simulink model "TPS"  (R2023b)
settings: Solver=FixedStepDiscrete  StartTime=0.0  StopTime=10.0  FixedStep=0.01  RelTol=1e-3
undefined symbols (not defined in the file or in its folder): MyEnum
settings Model: ExtModeTrigDuration=2  Creator=Beshary  LastModifiedBy=Beshary
settings OptimizationCC: DefaultParameterBehavior=Inlined  UseDivisionForNetSlopeComputation=on  GainParamInheritBuiltInType=on  UseFloatMulNetSlope=on  InlineInvariantSignals=on  PassReuseOutputArgsAs=Individual arguments  ZeroExternalMemoryAtStartup=off  ZeroInternalMemoryAtStartup=off  NoFixptDivByZeroProtection=on  EfficientFloat2IntCast=on  LifeSpan=1  MaxStackSize=64  OptimizeBlockOrder=speed  DifferentSizesBufferReuse=on  EfficientTunableParamExpr=on
settings DebuggingCC: ParameterTunabilityLossMsg=error
settings HardwareCC: ProdBitPerInt=16  ProdBitPerPointer=16  ProdBitPerSizeT=16  ProdBitPerPtrDiffT=16  ProdLargestAtomicFloat=None  ProdWordSize=8  ProdLongLongMode=on  ProdHWDeviceType=Atmel->AVR
settings SFSimCC: MATLABDynamicMemAlloc=off
settings RTWCC: Description=Embedded Coder  SystemTargetFile=ert.tlc  HardwareBoard=Arduino Uno  TemplateMakefile=ert_default_tmf  Toolchain=Arduino AVR  BuildConfiguration=Faster Runs
settings CodeAppCC: ForceParamTrailComments=on  IgnoreCustomStorageClasses=off  OperatorAnnotations=on  SimulinkDataObjDesc=on  SFDataObjDesc=on  CustomSymbolStrGlobalVar=rt$N$M  CustomSymbolStrType=$N$M  CustomSymbolStrFcn=$N$M$F  CustomSymbolStrMacro=$N$M  InsertBlockDesc=on
settings ERTTargetCC: IncludeMdlTerminateFcn=off  CombineSignalStateStructs=on  SuppressErrorStatus=on  SupportAbsoluteTime=off  SupportComplex=off  ExtModeTransport=3  ExtModeStaticAlloc=on  ExtModeAutomaticAllocSize=off  ExtModeStaticAllocSize=250  ExtModeMexFile=ext_xcp  ExtModeIntrfLevel=Level2 - Open  InlinedParameterPlacement=NonHierarchical  ERTFilePackagingFormat=CompactWithDataFile

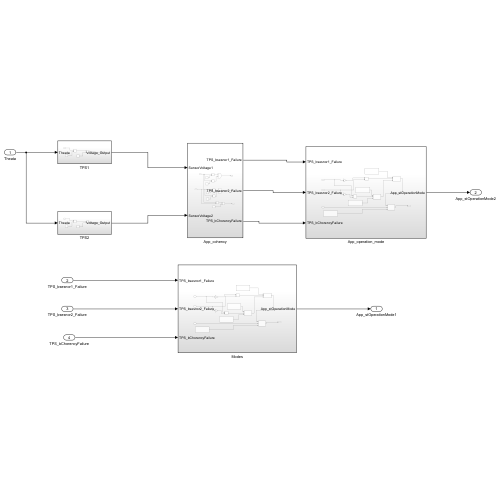
[thumbnail: Simulink's stored preview of the top-level diagram]
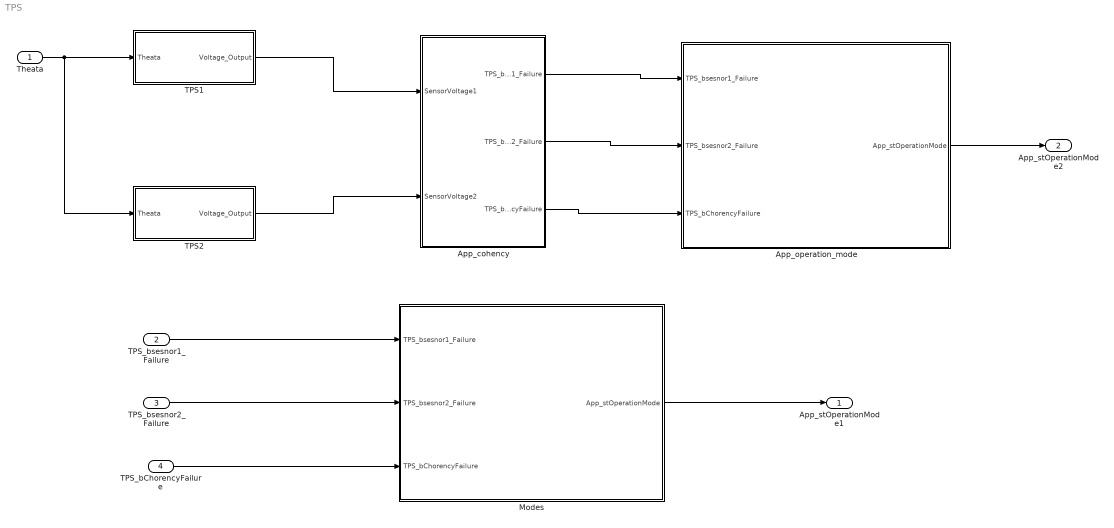
== system TPS ==
  Theata : Inport
  TPS_bsesnor1_Failure : Inport  Port=2
  TPS_bsesnor2_Failure : Inport  Port=3
  TPS_bChorencyFailure : Inport  Port=4
  App_cohency : Subsystem
  App_operation_mode : Subsystem
  Modes : Subsystem
  TPS1 : Subsystem
  TPS2 : Subsystem
  App_stOperationMode1 : Outport
  App_stOperationMode2 : Outport  Port=2
  wires:
  Theata/1 -> TPS2/1(Theata), TPS1/1(Theata)
  TPS1/1(Voltage_Output) -> App_cohency/1(SensorVoltage1)
  TPS2/1(Voltage_Output) -> App_cohency/2(SensorVoltage2)
  App_cohency/1(TPS_bsesnor1_Failure) -> App_operation_mode/1(TPS_bsesnor1_Failure)
  App_cohency/2(TPS_bsesnor2_Failure) -> App_operation_mode/2(TPS_bsesnor2_Failure)
  App_cohency/3(TPS_bChorencyFailure) -> App_operation_mode/3(TPS_bChorencyFailure)
  App_operation_mode/1(App_stOperationMode) -> App_stOperationMode2/1
  TPS_bChorencyFailure/1 -> Modes/3(TPS_bChorencyFailure)
  TPS_bsesnor2_Failure/1 -> Modes/2(TPS_bsesnor2_Failure)
  TPS_bsesnor1_Failure/1 -> Modes/1(TPS_bsesnor1_Failure)
  Modes/1(App_stOperationMode) -> App_stOperationMode1/1

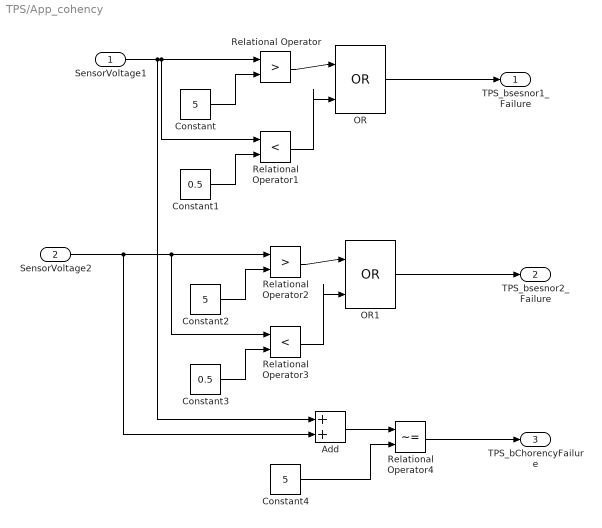
== system TPS/App_cohency ==
  SensorVoltage1 : Inport
  SensorVoltage2 : Inport  Port=2
  Add : Sum
  Constant : Constant  Value=5
  Constant1 : Constant  Value=0.5
  Constant2 : Constant  Value=5
  Constant3 : Constant  Value=0.5
  Constant4 : Constant  Value=5
  OR : Logic  Operator=OR  IconShape=distinctive  AllPortsSameDT=off  OutDataTypeStr=boolean
  OR1 : Logic  Operator=OR  IconShape=distinctive  AllPortsSameDT=off  OutDataTypeStr=boolean
  Relational Operator : RelationalOperator  Operator=>  OutDataTypeStr=boolean  RndMeth=Simplest  InputSameDT=off
  Relational Operator1 : RelationalOperator  Operator=<  OutDataTypeStr=boolean  RndMeth=Simplest  InputSameDT=off
  Relational Operator2 : RelationalOperator  Operator=>  OutDataTypeStr=boolean  RndMeth=Simplest  InputSameDT=off
  Relational Operator3 : RelationalOperator  Operator=<  OutDataTypeStr=boolean  RndMeth=Simplest  InputSameDT=off
  Relational Operator4 : RelationalOperator  Operator=~=  OutDataTypeStr=boolean  RndMeth=Simplest  InputSameDT=off
  TPS_bsesnor1_Failure : Outport
  TPS_bsesnor2_Failure : Outport  Port=2
  TPS_bChorencyFailure : Outport  Port=3
  wires:
  Constant/1 -> Relational Operator/2
  Relational Operator/1 -> OR/1
  Constant1/1 -> Relational Operator1/2
  SensorVoltage1/1 -> Add/1, Relational Operator1/1, Relational Operator/1
  Relational Operator1/1 -> OR/2
  OR/1 -> TPS_bsesnor1_Failure/1
  Relational Operator3/1 -> OR1/2
  SensorVoltage2/1 -> Add/2, Relational Operator2/1, Relational Operator3/1
  Constant3/1 -> Relational Operator3/2
  Relational Operator2/1 -> OR1/1
  Constant2/1 -> Relational Operator2/2
  OR1/1 -> TPS_bsesnor2_Failure/1
  Add/1 -> Relational Operator4/1
  Constant4/1 -> Relational Operator4/2
  Relational Operator4/1 -> TPS_bChorencyFailure/1

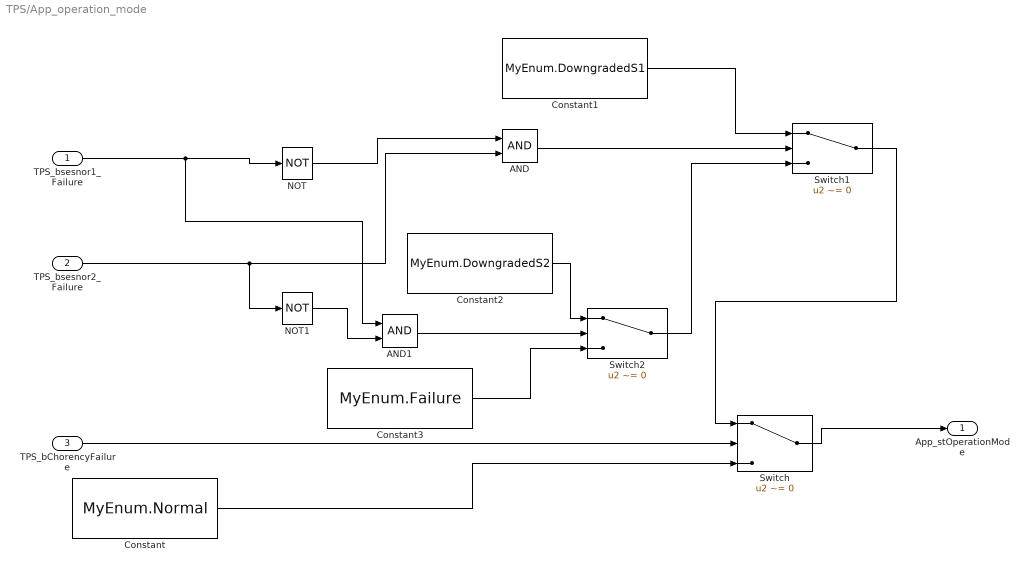
== system TPS/App_operation_mode ==
  TPS_bsesnor1_Failure : Inport
  TPS_bsesnor2_Failure : Inport  Port=2
  TPS_bChorencyFailure : Inport  Port=3
  AND : Logic  AllPortsSameDT=off  OutDataTypeStr=boolean
  AND1 : Logic  AllPortsSameDT=off  OutDataTypeStr=boolean
  Constant : Constant  Value=MyEnum.Normal
  Constant1 : Constant  Value=MyEnum.DowngradedS1
  Constant2 : Constant  Value=MyEnum.DowngradedS2
  Constant3 : Constant  Value=MyEnum.Failure
  NOT : Logic  Operator=NOT  IconShape=distinctive  AllPortsSameDT=off  OutDataTypeStr=boolean
  NOT1 : Logic  Operator=NOT  IconShape=distinctive  AllPortsSameDT=off  OutDataTypeStr=boolean
  Switch : Switch  Criteria=u2 ~= 0  SaturateOnIntegerOverflow=off  InputSameDT=off
  Switch1 : Switch  Criteria=u2 ~= 0  SaturateOnIntegerOverflow=off  InputSameDT=off
  Switch2 : Switch  Criteria=u2 ~= 0  SaturateOnIntegerOverflow=off  InputSameDT=off
  App_stOperationMode : Outport  OutDataTypeStr=Enum: MyEnum
  wires:
  TPS_bChorencyFailure/1 -> Switch/2
  Constant/1 -> Switch/3
  Switch/1 -> App_stOperationMode/1
  TPS_bsesnor1_Failure/1 -> AND1/1, NOT/1
  NOT/1 -> AND/1
  TPS_bsesnor2_Failure/1 -> NOT1/1, AND/2
  AND/1 -> Switch1/2
  Switch1/1 -> Switch/1
  Constant1/1 -> Switch1/1
  NOT1/1 -> AND1/2
  AND1/1 -> Switch2/2
  Constant2/1 -> Switch2/1
  Constant3/1 -> Switch2/3
  Switch2/1 -> Switch1/3

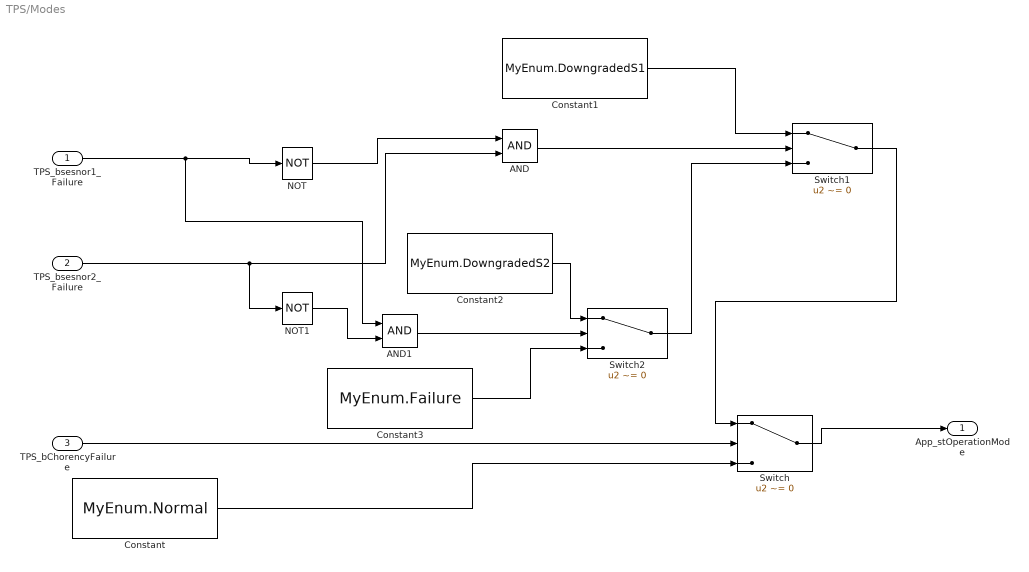
== system TPS/Modes ==
  TPS_bsesnor1_Failure : Inport
  TPS_bsesnor2_Failure : Inport  Port=2
  TPS_bChorencyFailure : Inport  Port=3
  AND : Logic  AllPortsSameDT=off  OutDataTypeStr=boolean
  AND1 : Logic  AllPortsSameDT=off  OutDataTypeStr=boolean
  Constant : Constant  Value=MyEnum.Normal
  Constant1 : Constant  Value=MyEnum.DowngradedS1
  Constant2 : Constant  Value=MyEnum.DowngradedS2
  Constant3 : Constant  Value=MyEnum.Failure
  NOT : Logic  Operator=NOT  IconShape=distinctive  AllPortsSameDT=off  OutDataTypeStr=boolean
  NOT1 : Logic  Operator=NOT  IconShape=distinctive  AllPortsSameDT=off  OutDataTypeStr=boolean
  Switch : Switch  Criteria=u2 ~= 0  SaturateOnIntegerOverflow=off  InputSameDT=off
  Switch1 : Switch  Criteria=u2 ~= 0  SaturateOnIntegerOverflow=off  InputSameDT=off
  Switch2 : Switch  Criteria=u2 ~= 0  SaturateOnIntegerOverflow=off  InputSameDT=off
  App_stOperationMode : Outport  OutDataTypeStr=Enum: MyEnum
  wires:
  Switch2/1 -> Switch1/3
  Constant3/1 -> Switch2/3
  Constant2/1 -> Switch2/1
  AND1/1 -> Switch2/2
  NOT1/1 -> AND1/2
  Constant1/1 -> Switch1/1
  Switch1/1 -> Switch/1
  AND/1 -> Switch1/2
  TPS_bsesnor2_Failure/1 -> AND/2, NOT1/1
  NOT/1 -> AND/1
  TPS_bsesnor1_Failure/1 -> NOT/1, AND1/1
  Switch/1 -> App_stOperationMode/1
  Constant/1 -> Switch/3
  TPS_bChorencyFailure/1 -> Switch/2

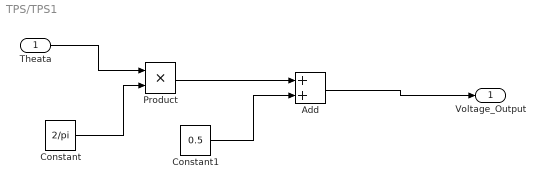
== system TPS/TPS1 ==
  Theata : Inport
  Add : Sum
  Constant : Constant  Value=2/pi
  Constant1 : Constant  Value=0.5
  Product : Product
  Voltage_Output : Outport
  wires:
  Constant/1 -> Product/2
  Product/1 -> Add/1
  Theata/1 -> Product/1
  Constant1/1 -> Add/2
  Add/1 -> Voltage_Output/1

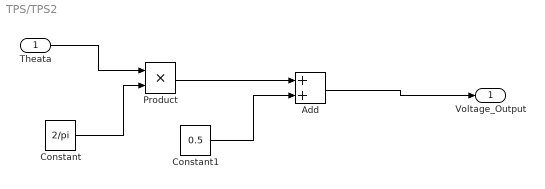
== system TPS/TPS2 ==
  Theata : Inport
  Add : Sum
  Constant : Constant  Value=2/pi
  Constant1 : Constant  Value=0.5
  Product : Product
  Voltage_Output : Outport
  wires:
  Add/1 -> Voltage_Output/1
  Constant1/1 -> Add/2
  Theata/1 -> Product/1
  Product/1 -> Add/1
  Constant/1 -> Product/2
